simulink subsystem "PvtSubSys_VSM_LCKIE"  (R2020b)
settings: Solver=VariableStepAuto  StartTime=0.0  StopTime=10.0  RelTol=1e-3
values from neighbouring files (symbols this model uses):
  P_VSM_LCKIE_ClassInput = 0.0    [LCKIE.sldd]
  P_VSM_LCKIE_Laneoffset : value not decoded    [LCKIE.sldd]
  P_VSM_LCKIE_Laneoffset_BP : value not decoded    [LCKIE.sldd]
  P_VSM_LCKIE_LatC_DisOffofLanWidth : value not decoded    [LCKIE.sldd]
  P_VSM_LCKIE_LatC_DisOffofSpd : value not decoded    [LCKIE.sldd]
  P_VSM_LCKIE_LatC_DisSW = 0.0    [LCKIE.sldd]
  P_VSM_LCKIE_LatC_LanWidth : value not decoded    [LCKIE.sldd]
  P_VSM_LCKIE_LATC_LimitDis : value not decoded    [LCKIE.sldd]
  P_VSM_LCKIE_LATC_LimitDis_BP : value not decoded    [LCKIE.sldd]
  P_VSM_LCKIE_LatC_LimitDisEgoToObjSelt = 1.5    [LCKIE.sldd]
  P_VSM_LCKIE_LatC_LimitEgoToOppLane = 0.3    [LCKIE.sldd]
  P_VSM_LCKIE_LatC_maxLimitDisREToLane = 2.5    [LCKIE.sldd]
  P_VSM_LCKIE_LatC_minLimitDisREToLane = 1.2    [LCKIE.sldd]
  P_VSM_LCKIE_LatC_MoveEnableDis = 0.0    [LCKIE.sldd]
  P_VSM_LCKIE_LatC_RESafDis = 0.8    [LCKIE.sldd]
  P_VSM_LCKIE_LatC_SafeDisofLanWidth : value not decoded    [LCKIE.sldd]
  P_VSM_LCKIE_LatC_Spd : value not decoded    [LCKIE.sldd]
  P_VSM_LCKIE_LongC_d1 : value not decoded    [LCKIE.sldd]
  P_VSM_LCKIE_LongC_d2 : value not decoded    [LCKIE.sldd]
  P_VSM_LCKIE_LongC_DetaSpd : value not decoded    [LCKIE.sldd]
  P_VSM_LCKIE_LongC_DirecChangeDis = 20.0    [LCKIE.sldd]
  P_VSM_LCKIE_LongC_FleetOff = 80.0    [LCKIE.sldd]
  P_VSM_LCKIE_LongC_maxDis = 80.0    [LCKIE.sldd]
  P_VSM_LCKIE_LongC_minDis = 50.0    [LCKIE.sldd]
  P_VSM_LCKIE_LongC_ShutDownLongDis = -25.0    [LCKIE.sldd]
  P_VSM_LCKIE_LongC_ShutDownTTC = -4.0    [LCKIE.sldd]
  P_VSM_LCKIE_LongC_Spd : value not decoded    [LCKIE.sldd]
  P_VSM_LCKIE_LongC_toff = 10.0    [LCKIE.sldd]
  P_VSM_LCKIE_OFC_ActDis = 10.0    [LCKIE.sldd]
  P_VSM_LCKIE_OFC_DownDis = 10.0    [LCKIE.sldd]
  P_VSM_LCKIE_OFC_DownTTC = 5.0    [LCKIE.sldd]
  P_VSM_LCKIE_OFC_SafDis = 10.0    [LCKIE.sldd]
  P_VSM_LCKIE_OFC_Toff = 3.0    [LCKIE.sldd]
  P_VSM_LCKIE_ORC_LatDis = 1.8    [LCKIE.sldd]
  P_VSM_LCKIE_ORC_LimitDis1 = -30.0    [LCKIE.sldd]
  P_VSM_LCKIE_ORC_LimitDis2 = -10.0    [LCKIE.sldd]
  P_VSM_LCKIE_ORC_LimitTTC = 10.0    [LCKIE.sldd]
  P_VSM_LCKIE_ORC_LowSpd = -5.0    [LCKIE.sldd]
  P_VSM_LCKIE_POC_Delaytime : value not decoded    [LCKIE.sldd]
  P_VSM_LCKIE_POC_detaSpd : value not decoded    [LCKIE.sldd]
  P_VSM_LCKIE_POC_LimitDis = -15.0    [LCKIE.sldd]
  P_VSM_LCKIE_POC_LimitTTC = 2.0    [LCKIE.sldd]
  P_VSM_LCKIE_State_CurveMax = 0.005    [LCKIE.sldd]
  P_VSM_LCKIE_State_CurveMin = 0.0055555555555555558    [LCKIE.sldd]
  P_VSM_LCKIE_State_detaspd = 1.39    [LCKIE.sldd]
  P_VSM_LCKIE_State_detaspd_enable = 1.0    [LCKIE.sldd]
  P_VSM_LCKIE_State_DriverInputTrqValue_enable = 1.0    [LCKIE.sldd]
  P_VSM_LCKIE_State_ELKObjClc = 1.0    [LCKIE.sldd]
  P_VSM_LCKIE_State_HWASts_disable = 1.0    [LCKIE.sldd]
  P_VSM_LCKIE_State_IEObjClc = 1.0    [LCKIE.sldd]
  P_VSM_LCKIE_State_IFVReady = 1.0    [LCKIE.sldd]
  P_VSM_LCKIE_State_lamb_enable = 1.0    [LCKIE.sldd]
  P_VSM_LCKIE_State_Lanecurve_enable = 1.0    [LCKIE.sldd]
  P_VSM_LCKIE_State_LaneWidth_enable = 1.0    [LCKIE.sldd]
  P_VSM_LCKIE_State_Off2on = 3.0    [LCKIE.sldd]
  P_VSM_LCKIE_State_OppObjClc = 1.0    [LCKIE.sldd]
  P_VSM_LCKIE_STATE_ORCObjenable = 0.0    [LCKIE.sldd]
  P_VSM_LCKIE_State_Vehspeed_enable = 1.0    [LCKIE.sldd]
  P_VSM_LCKIE_State_wiper_enable = 1.0    [LCKIE.sldd]
  P_VSM_LCKIE_tcycle = 0.02    [LCKIE.sldd]
undefined symbols (not defined in the file or in its folder): P_Global_Vehicle_Length_m, P_Global_VehicleWidthMin_m, P_VSM_LSMC_SampleTime, STATE
libraries: simulink x62
(part 4 of 5)

== system PvtSubSys_VSM_LCKIE/LCKIE/Subsystem1/LCKIE_SignalProcess1/IE_POC/Subsystem ==
  Input : Inport
  Add : Sum  Inputs=++++++
  Gain : Gain  Gain=1/6
  Unit Delay{,2,4..6} (5 alike) : UnitDelay  SampleTime=-1  HasFrameUpgradeWarning=on
  Out1 : Outport
  wires:
  Input/1 -> Unit Delay6/1, Unit Delay5/1, Unit Delay/1, Unit Delay4/1, Unit Delay2/1, Add/1
  Add/1 -> Gain/1
  Unit Delay4/1 -> Add/3
  Unit Delay/1 -> Add/4
  Gain/1 -> Out1/1
  Unit Delay6/1 -> Add/6
  Unit Delay2/1 -> Add/2
  Unit Delay5/1 -> Add/5

== matlab function PvtSubSys_VSM_LCKIE/LCKIE/LCKIE_StateMachine/Subsystem1/MATLAB Function ==
  data: DisLimmit input single; Dis output single; slope input single; DisK1 input single
function Dis = fcn(DisLimmit,slope,DisK1)
Dis = DisK1;
if DisLimmit >=0
    if (DisK1 - slope <= DisLimmit )&& (DisLimmit <= DisK1 + slope)
        Dis = DisLimmit;
    elseif DisK1 > DisLimmit - slope
        Dis = Dis - slope;
    elseif DisK1 < DisLimmit - slope
        Dis = Dis + slope;
    end
else
    if (DisK1 - slope <= DisLimmit )&& (DisLimmit <= DisK1 + slope)
        Dis = DisLimmit;        
    elseif DisK1 > DisLimmit + slope
        Dis = Dis - slope;
    elseif DisK1 < DisLimmit + slope
        Dis = Dis + slope;
    end
end

== matlab function PvtSubSys_VSM_LCKIE/LCKIE/Subsystem1/IEStateClc/MATLAB Function1 ==
  data: HWASts input uint8; LCKSts input; LaneChange input boolean; Flg output uint8; reflgK1 input uint8; reflg output uint8
function [Flg,reflg]  = fcn(HWASts,LCKSts,LaneChange,reflgK1)
Flg = uint8(0);
reflg = uint8(0);

if LCKSts == 3   
    Flg = uint8(1);
    if (HWASts == 5 ||HWASts == 6)
        Flg = uint8(0);
        if LaneChange == 1
            Flg = uint8(1);
            reflg = uint8(1);
        end
        if reflgK1 == 1
            Flg = uint8(1);
            reflg = uint8(1);
        end
    end
end

== matlab function PvtSubSys_VSM_LCKIE/LCKIE/Subsystem1/LCKIE_SignalProcess1/IE_LATC/MATLAB Function1 ==
  data: Direct input uint8; latflg input uint8; latmov input single; movdis output single; detaDis output; Dis2Obj input single; ORCID input uint8; SelctID input uint8; ORCReady input uint8; ORCReadyK1 input; IEAct input; limitDis input single; flgK1 input uint8; flg output uint8
function [movdis,detaDis,flg] = fcn(Direct,latflg,latmov,Dis2Obj,ORCID,SelctID,ORCReady,ORCReadyK1,IEAct,limitDis,flgK1)

detaDis = single(0);
movdis = latmov;
flg = uint8(0);
if IEAct==1
    flg = flgK1;
    if ORCReady==0 && (ORCReadyK1==1 ||flgK1==1)
        flg = uint8(1);
    end
    if ORCReady==1 && ORCReadyK1==0 
        flg = uint8(0);
    end
end

if flg==1
    t_s = round((Dis2Obj(ORCID)+Dis2Obj(SelctID))*5)/10;
    if latflg == 1
        if abs(t_s)<latmov
            if Direct==1 && t_s<0
                movdis = latmov +t_s;
            elseif Direct==1 && t_s >0
                movdis = latmov - t_s;
            end
        else
            if Direct==1
                if t_s > 0
                    movdis = latmov;
                else
                    detaDis = abs(t_s + latmov);
                    movdis = limitDis;
                end
            else
                if t_s < 0
                    movdis = latmov;
                else
                    detaDis = abs(t_s - latmov);
                    movdis = limitDis;
                end
            end
        end
    end
end

== matlab function PvtSubSys_VSM_LCKIE/LCKIE/Subsystem1/LCKIE_SignalProcess1/IE_Long/IE_LongClc ==
  data: DirectChange input uint8; LongDis output single; PocFlg output uint8; IEReady output uint8; LongFlg output uint8; CouterOff output uint16; ID output uint8; Counter output uint8; Counter1 output uint16 size=1; Counter2 output uint16 size=1; Counter3 output uint16 size=1; Dx output single; LatFLg input uint8; ObjLatFailFlg input uint8; TTC input single; ObjSelectID input uint8; DetaSpdSelct input single; ObjLongPos input single; ObjID input uint8; POSLaneRObjID input uint8; LongDown input uint8; time_shutdown input single; LongDisClc input single; FleetOff input single; ShutDownTTC input single; ShutDownLongDis input single; minDis input single; maxDis input single; DirecChangeDis input single; t_LongDis input single; t_cycle input single; IEActK1 input boolean; LongFlgK1 input uint8; CouterOffK1 input uint16; IDK1 input uint8; CounterK1 input uint8; Counter1K1 input uint16; Counter2K1 input uint16; Counter3K1 input uint16; DxK1 input single
function [LongDis,PocFlg,IEReady,LongFlg,CouterOff,ID,Counter,Counter1,Counter2,Counter3,Dx] = fcn(DirectChange,LatFLg,ObjLatFailFlg,...
    TTC,ObjSelectID,DetaSpdSelct,ObjLongPos,ObjID,POSLaneRObjID,LongDown,...
    time_shutdown,LongDisClc,FleetOff,ShutDownTTC,ShutDownLongDis,minDis,maxDis,DirecChangeDis,t_LongDis,t_cycle,...
    IEActK1,LongFlgK1,CouterOffK1,IDK1,CounterK1,Counter1K1,Counter2K1,Counter3K1,DxK1)


ID = uint8(0);
ObjRPosLanelong = single(0);
ObjRPosLaneTTC = single(0);
SpdLimit = single(0);
LongFlg = uint8(0);
PocFlg = uint8(0);
IEReady = uint8(0);
Counter = uint8(0);
Counter1 = uint16(0);
Counter2 = uint16(0);
Counter3 = uint16(0);
CouterOff = CouterOffK1;
LongDis = LongDisClc;
Dx = single(0);


if ObjSelectID >0
    Dx = ObjLongPos(ObjSelectID);
    ID = ObjID(ObjSelectID);
end
if ID == IDK1
    SpdLimit = single(-2);
end

if POSLaneRObjID >0
    ObjRPosLanelong =  ObjLongPos(POSLaneRObjID);
    ObjRPosLaneTTC =  TTC(POSLaneRObjID);
end



if IEActK1 < 1
    CouterOff = uint16(0);
    if  LongDis > 0 && ObjSelectID >0
        if LongFlgK1 == 0
            if Dx<= LongDis
                Counter = min(CounterK1+uint8(1),uint8(50));
                if Counter > 10
                    LongFlg = uint8(1);
                end
            end
        else
            if ID == IDK1  %%纵向Flg锁
                LongDis = FleetOff;
                if Dx<= LongDis
                    LongFlg = uint8(1);
                end
            end
        end
    end
else
    if ObjSelectID == 0  %%退出机制
        if IDK1 ~= 0 
            LongFlg = uint8(1);            
            if DxK1 >=20  %%防止目标纵向距离跳变
                CouterOff = uint16(100);
            else
                CouterOff = uint16(time_shutdown /t_cycle);
            end
        else
            PocFlg = uint8(1);
            if POSLaneRObjID > 0  %%常规退出条件
                if ObjRPosLaneTTC < ShutDownTTC && ObjRPosLanelong < ShutDownLongDis
                    LongFlg = uint8(0);
                else
                    LongFlg = uint8(1);
                end
            else
                Counter1 = min((Counter1K1+uint16(1)),uint16(65534));                               
                if Counter1 < CouterOff
                    LongFlg = uint8(1);
                end                
            end
        end
    else
        CouterOff = uint16(time_shutdown /t_cycle);
        d3 = DetaSpdSelct*t_LongDis;
        t_d = min(max(d3,minDis),maxDis);        
        LongDis = t_d;
        if DirectChange ==0
            if Dx<= LongDis  && DetaSpdSelct > SpdLimit
                LongFlg = uint8(1);
            else
                PocFlg = uint8(1); 
                if POSLaneRObjID > 0
                    if ObjRPosLaneTTC < ShutDownTTC && ObjRPosLanelong < ShutDownLongDis
                        LongFlg = uint8(0);
                    else
                        LongFlg = uint8(1);
                    end
                else
                    if IDK1 == 0
                        Counter2 = min(max(Counter1K1,Counter2K1)+uint16(1),uint16(65534));                     
                    else
                        Counter2 = min(Counter2K1+uint16(1),uint16(65534));
                    end
            
                    if Counter2 < CouterOff
                        LongFlg = uint8(1);
                    end                   
                end
            end
        else
            LongDis = LongDis - DirecChangeDis;
            if Dx > LongDis && (TTC(ObjSelectID)>5 || DetaSpdSelct <0)
               PocFlg = uint8(1);
               if POSLaneRObjID > 0
                   if ObjRPosLaneTTC < ShutDownTTC && ObjRPosLanelong < ShutDownLongDis
                       LongFlg = uint8(0);
                   else
                       LongFlg = uint8(1);
                   end
               else
                   if IDK1 == 0
                       Counter3 = min(max(Counter1K1,Counter3K1)+uint16(1),uint16(65534));
                   else
                       Counter3 = min(Counter3K1+uint16(1),uint16(65534));
                   end                 
                   if Counter3 < CouterOff
                       LongFlg = uint8(1);
                   end                  
               end
           else
                LongFlg = uint8(0);
                ID = uint8(254);
           end
        end
    end
end

if LongDown ==1 && PocFlg ==1 
    LongFlg = uint8(0);
end

if IEActK1 == 0
    if LongFlg == 1 && LatFLg == 1
        IEReady = uint8(1);
    end
elseif IEActK1 ==1
    if LongFlg == 1 && ObjLatFailFlg ==0
        IEReady = uint8(1);
    end
end

== matlab function PvtSubSys_VSM_LCKIE/LCKIE/Subsystem1/LCKIE_SignalProcess1/IE_OFC/OFC2 ==
  data: safeDis input single; ActDis input single; Toff input single; T1 input single; Dis1 input single; EgoLong input single; OppLaneFObjID input uint8; DetaSpd input single; TTC input single; ObjLongPos input single; ObjLength input single; ObjSelsctDx output single size=1; OppObjDetaSpd output single size=1; ObjTTC output single; Tset output single; OppObjReady output uint8 size=1; OppObjFail output uint8; OppObjReadyK1 input uint8; OppObjFailK1 input uint8; CounterK1 input uint8; Counter output uint8 size=1; Counter1K1 input uint8; Counter1 output uint8
function [ObjSelsctDx,OppObjDetaSpd,ObjTTC,Tset,OppObjReady,OppObjFail,Counter,Counter1]= fcn(safeDis,ActDis,...
    Toff,T1,Dis1,EgoLong,OppLaneFObjID,DetaSpd,TTC,ObjLongPos,ObjLength,OppObjReadyK1,OppObjFailK1,CounterK1,Counter1K1)



OppObjReady = uint8(0);
ObjSelsctDx = single(0);
Counter = uint8(0);
Counter1 = uint8(0);
OppObjDetaSpd =single(0);
ObjLong = single(0);
ObjTTC=single(0);
Tset = single(0);
OppObjFail = uint8(0);

if OppLaneFObjID > 0
    ObjSelsctDx = single(ObjLongPos(OppLaneFObjID)-single(EgoLong));   
    OppObjDetaSpd = single(DetaSpd(OppLaneFObjID));  
    ObjTTC = TTC(OppLaneFObjID);
    if  ObjLength(OppLaneFObjID) ==0
        ObjLong = single(8);
    else
        ObjLong = max(min(ObjLength(OppLaneFObjID),single(20)),single(8));
    end

end

if OppLaneFObjID == 0 || ObjSelsctDx>=120
    OppObjReady = uint8(1);
else
   if  OppObjDetaSpd <0 && ObjSelsctDx>=8
        OppObjReady = uint8(1);
   else
       t_h = (ObjLong+2*safeDis)/OppObjDetaSpd;
       Tset =  Toff+t_h;
       if ObjTTC >Tset && ObjSelsctDx > ActDis
           OppObjReady = uint8(1);
       end
   end
end

if OppLaneFObjID > 0 && OppObjDetaSpd >0
  if (ObjTTC>0 && ObjTTC <T1)|| ObjSelsctDx < Dis1
      OppObjFail = uint8(1);
  end
end
    
if OppObjReady~= OppObjReadyK1
    Counter = min(CounterK1+uint8(1),uint8(20));
    if Counter < 15
        OppObjReady = OppObjReadyK1;
    end
end

if OppObjFail~= OppObjFailK1
    Counter1 = min(Counter1K1+uint8(1),uint8(20));
    if Counter1 < 15
        OppObjFail= OppObjFailK1;
    end
end

== matlab function PvtSubSys_VSM_LCKIE/LCKIE/Subsystem1/LCKIE_SignalProcess1/IE_ORC/ORC ==
  data: Dis1 input single; Dis2 input single; minTTC input single; LatDis input single; LowSpd input single; ObjSelsctTTC output single; OppLaneRObjID input uint8; ObjSelsctDx output single; OppObjLatDis output; OppObjSpd output single; DetaSpd input single; TTC input single; DisEgo2Obj input single; ObjLongPos input single; OppREARObjReadyK1 input uint8; CouterK1 input uint8; OppREARObjReady output uint8; Couter output uint8
function [ObjSelsctTTC,ObjSelsctDx,OppObjLatDis,OppObjSpd,...
    OppREARObjReady,Couter]= fcn(Dis1,Dis2,minTTC,LatDis,LowSpd,OppLaneRObjID,...
    DetaSpd,TTC,DisEgo2Obj,ObjLongPos,OppREARObjReadyK1,CouterK1)



OppREARObjReady = uint8(0);
ObjSelsctDx = single(0);
OppObjSpd =single(0);
ObjSelsctTTC = single(0);
OppObjLatDis = single(0);
Couter = uint8(0);


if OppLaneRObjID > 0
    ObjSelsctDx = single(ObjLongPos(OppLaneRObjID));   
    OppObjLatDis = abs(single(DisEgo2Obj(OppLaneRObjID)));  
    OppObjSpd = single(DetaSpd(OppLaneRObjID));
    ObjSelsctTTC = single(TTC(OppLaneRObjID));
end
if OppLaneRObjID == 0 
    OppREARObjReady = uint8(1);
else
    if OppObjSpd < 0  && OppObjSpd > LowSpd 
        if ObjSelsctDx < Dis1 && ObjSelsctTTC < minTTC && OppObjLatDis > LatDis
            OppREARObjReady = uint8(1);
        end
    else
        if ObjSelsctDx < Dis2
            OppREARObjReady = uint8(1);
        end
    end
end

if OppREARObjReady ~= OppREARObjReadyK1
    Couter = min(CouterK1 +uint8(1),uint8(15));
    if Couter<10
        OppREARObjReady = OppREARObjReadyK1;
    end
end

== matlab function PvtSubSys_VSM_LCKIE/LCKIE/Subsystem1/LCKIE_SignalProcess1/IE_OS/OS ==
  data: IEACTK1 input boolean; IEState input uint8; ObjNum input uint8; t_Ego2Left input single; t_Ego2Right input single; ObjID input uint8; OppFObjID output uint8; ObjLongPos input single; ObjLatPos input single; ObjWidth input single; ObjFuType input uint8; ObjVx input single; ObjClass input uint8; VheSpd_ms input single; C_valid input boolean; C_A0 input single; C_A1 input single; C_A2 input single; C_A3 input single; L_valid input boolean; L_A0 input single; L_A1 input single; L_A2 input single; L_A3 input single; R_valid input boolean; R_A0 input single; R_A1 input single; R_A2 input single; R_A3 input single; ObjIDSelectK1 input uint8; CouterK1 input uint8; Couter1K1 input uint8; OppRObjID output uint8; POSRObjID output uint8; DisEgo2ObjSelect output single; DisEgoToObj output; DetaSpdSelect output single; DisEgo2OppLane output single; DetaSpd output single; ObjLane output uint8; TTC output single; ObjSelectID output uint8; ObjIDSelect output uint8; Couter output uint8; Couter1 output uint8
function [OppFObjID,OppRObjID,POSRObjID,DisEgo2ObjSelect,DisEgoToObj,DetaSpdSelect,DisEgo2OppLane,DetaSpd,ObjLane,TTC,...
    ObjSelectID,ObjIDSelect,Couter,Couter1] = fcn(IEACTK1,IEState,ObjNum,t_Ego2Left,t_Ego2Right,ObjID,...
    ObjLongPos,ObjLatPos,ObjWidth,ObjFuType,ObjVx,ObjClass,VheSpd_ms,C_valid,C_A0,C_A1,C_A2,C_A3,...
    L_valid,L_A0,L_A1,L_A2,L_A3,R_valid,R_A0,R_A1,R_A2,R_A3,ObjIDSelectK1,CouterK1,Couter1K1)

ObjLane = uint8(zeros(9,1));
DetaSpd = single(zeros(9,1));
TTC = single(255*zeros(9,1));
DisEgoToObj = single(255*zeros(9,1));
OppFObjID = uint8(0);
OppRObjID = uint8(0);
POSRObjID = uint8(0);
DisEgo2ObjSelect = single(0);
DetaSpdSelect =  single(0);
DisEgo2OppLane =  single(0);
ObjSelectID = uint8(0);
ObjIDSelect = uint8(0);
Couter = uint8(0);
Couter1 = uint8(0);

minLFObjDis = single(255);
minRFObjDis = single(255);
minEgoFDis = single(255);
minLFTruckDis = single(255);
minRFTruckDis = single(255);
minLRDis = single(255);
minRRDis = single(255);
minLFObjID = uint8(0);
minRFObjID = uint8(0);
minEgoFID = uint8(0);
minLFTruckID = uint8(0);
minRFTruckID = uint8(0);
minLRID = uint8(0);
minRRID = uint8(0);

for i=1:ObjNum
    %%
    if ObjID(i) == ObjIDSelectK1
        outoff = single(3.5);
        long1 = single(-110);
        long2 = single(130);
        LongSt = single(0);
        DirectSpd = single(-0.65);
    else
        outoff = single(3.3);
        long1 = single(-100);
        long2 = single(120);
        LongSt = single(1);
        DirectSpd = single(-0.25);
    end
    %% 目标属性提取，后方目标针对弯道情况，借用LM相关位置进行分类
    t_x = ObjLongPos(i);
    t_y = ObjLatPos(i);
    t_w = ObjWidth(i)/2;
    if ObjID(i) >0 && t_x >long1 &&  t_x < long2 && ObjFuType(i)~=2
        if t_x >LongSt  %%目标前后位置区分
            ObjLongSts = uint8(1);
        else
            ObjLongSts = uint8(2);
        end
        DetaSpd(i)= -ObjVx(i);
        absObjSpd = single(VheSpd_ms + ObjVx(i)); %%目标运动方向区分
        if absObjSpd > DirectSpd
            ObjMovDir = 1;
        else
            ObjMovDir = 2;
        end
        if abs(ObjVx(i)) > 0.001 %%TTC计算
            TTC(i) = -t_x/ObjVx(i);
        end
        if C_valid >0 && L_valid > 0 && R_valid > 0
            t_Cy = C_A0+C_A1*t_x+C_A2*t_x^2+C_A3*t_x^3;
            if t_y>t_Cy
                t_side = uint8(1); %% Obj in the left of ego vhicle
            else
                t_side = uint8(2);
            end
            if t_side == 1
                t_Ly = L_A0+L_A1*t_x+L_A2*t_x^2+L_A3*t_x^3;
                kL = L_A1+2*L_A2*t_x+3*L_A3*t_x^2;
                t_Lk = sqrt(kL^2+1);
                ObjEdge2Lane = (t_y - t_Ly)/t_Lk - t_w ;
            else
                t_Ry = R_A0+R_A1*t_x+R_A2*t_x^2+R_A3*t_x^3;
                kR = R_A1+2*R_A2*t_x+3*R_A3*t_x^2;
                t_Rk = sqrt(kR^2+1);
                ObjEdge2Lane = (t_Ry - t_y)/t_Rk - t_w ;
            end
            if ObjLongSts == 1
                t_latDis = ObjEdge2Lane + 0.4;
            else
                t_latDis = abs(ObjEdge2Lane);
            end
            if t_latDis <= 0
                ObjLane(i) = uint8(3);
            elseif t_latDis > 0 && t_latDis <= outoff
                if t_side ==1
                    ObjLane(i) = uint8(1);
                    DisEgoToObj(i) = t_Ego2Left + ObjEdge2Lane;
                elseif t_side ==2
                    ObjLane(i) = uint8(2);
                    DisEgoToObj(i) = -(t_Ego2Right + ObjEdge2Lane);
                end
            end
        end      
       
        if ObjLongSts == 1
            if ObjLane(i) == 1
                if minLFObjDis >= t_x
                    minLFObjDis = t_x;
                    minLFObjID = uint8(i);
                end
            elseif ObjLane(i) == 2
                if minRFObjDis >= t_x
                    minRFObjDis = t_x;
                    minRFObjID = uint8(i);
                end
            elseif ObjLane(i) == 3
                if minEgoFDis > t_x
                    minEgoFDis = t_x;
                    minEgoFID = uint8(i);
                end
            end
        end
        
        if ObjClass(i) ==3 && ObjLongSts == 1 && ObjMovDir == 1
            if ObjLane(i) == 1
                if minLFTruckDis >= t_x
                    minLFTruckDis = t_x;
                    minLFTruckID = uint8(i);
                end
            elseif ObjLane(i) == 2
                if minRFTruckDis >= t_x
                    minRFTruckDis = t_x;
                    minRFTruckID = uint8(i);
                end
            end
        end
        
        if ObjLongSts == 2 &&ObjMovDir == 1
            if ObjLane(i) == 1
                if minLRDis > abs(t_x)
                    minLRDis = abs(t_x);
                    minLRID = uint8(i);
                end
            elseif ObjLane(i) == 2
                if minRRDis> abs(t_x)
                    minRRDis = abs(t_x);
                    minRRID = uint8(i);
                end
            end
        end
    end
end
%% 主目标筛选，并针对相对速度进行相应延时选择处理
if minLFTruckID>0 && minRFTruckID >0
    t_h = minLFTruckDis - minRFTruckDis;
    if t_h >0
        t_selectID = minRFTruckID;
    else
        t_selectID = minLFTruckID;
    end
elseif minLFTruckID == 0 && minRFTruckID >0
    t_selectID = minRFTruckID;
elseif minLFTruckID > 0 && minRFTruckID == 0
    t_selectID = minLFTruckID;
else
    t_selectID = uint8(0);
end
if t_selectID >0
    if ObjID(t_selectID) == ObjIDSelectK1
        if DetaSpd(t_selectID) > -1.3
            ObjSelectID = t_selectID;
        else
            Couter = min(CouterK1+uint8(1),uint8(6));
            if Couter <5
                ObjSelectID = t_selectID;
            end
        end
    else
        if  DetaSpd(t_selectID) >0.1
            Couter1 = min(Couter1K1+uint8(1),uint8(16));
            if Couter1 >10
                ObjSelectID = t_selectID;
            end
        end
    end
end
%%
if ObjSelectID >0
    if ObjLane(ObjSelectID) == 1   
        DisEgo2OppLane = t_Ego2Right;
        OppFObjID = minRFObjID;
        OppRObjID = minRRID;
        POSRObjID = minLRID;
    elseif ObjLane(ObjSelectID) == 2
        DisEgo2OppLane = t_Ego2Left;
        OppFObjID = minLFObjID;
        OppRObjID = minLRID;
        POSRObjID = minRRID;
    end
else
    if IEACTK1==1
        if IEState == 5
            DisEgo2OppLane = t_Ego2Left;
            OppFObjID = minLFObjID;
            OppRObjID = minLRID;
            POSRObjID = minRRID;
        elseif IEState == 4
            DisEgo2OppLane = t_Ego2Right;
            OppFObjID = minRFObjID;
            OppRObjID = minRRID;
            POSRObjID = minLRID;
        end
    end
end
if ObjSelectID >0
    DisEgo2ObjSelect = abs(DisEgoToObj(ObjSelectID));
    DetaSpdSelect =  DetaSpd(ObjSelectID);
    ObjIDSelect = ObjID(ObjSelectID);
end

== matlab function PvtSubSys_VSM_LCKIE/LCKIE/Subsystem1/LCKIE_SignalProcess1/IE_LATC/LATC ==
  data: LatWarning output uint8; DirectChange output uint8; ObjLatFailFlg output uint8; MovDirct output uint8; LatFLg output uint8; IEActFlgK1 input boolean; ObjSelIDK1 input uint8; ObjSelID input uint8; ObjSelectID input uint8; DisEgo2ObjSelt input single; Ego2OppLane input single; DirctClc input uint8; MoveDis input single; MovDisK1 input single; DisEgo2oObjOff input single; minDisEgoToObjSelt input single; minEgoToOppLane input single; MoveEnableDis input single; MovDirctK1 input uint8; LatMovDis output single; LatFLgK1 input uint8; LatMovDisK1 input single; CounterK1 input uint8; Counter1K1 input uint8; Counter2K1 input uint8; Counter3K1 input uint8; Counter4K1 input uint8; Couter5K1 input uint8; Counter output uint8; Counter1 output uint8; Counter2 output uint8; Counter3 output uint8; Counter4 output uint8; Counter5 output uint8
function [LatWarning,DirectChange,ObjLatFailFlg,MovDirct,LatFLg,...
    LatMovDis,Counter,Counter1,Counter2,Counter3,Counter4,Counter5] = fcn(IEActFlgK1,ObjSelIDK1,ObjSelID,ObjSelectID,...
    DisEgo2ObjSelt,Ego2OppLane,DirctClc,MoveDis,MovDisK1,DisEgo2oObjOff,minDisEgoToObjSelt,minEgoToOppLane,MoveEnableDis,...
    MovDirctK1,LatFLgK1,LatMovDisK1,CounterK1,Counter1K1,Counter2K1,Counter3K1,Counter4K1,Couter5K1)

Counter = uint8(0);
Counter1 = uint8(0);
Counter2 = uint8(0);
Counter3 = uint8(0);
Counter4 = uint8(0);
Counter5 = uint8(0);
LatFLg = uint8(0);
LatMovDis = single(0);
DirectChange = uint8(0);
LatWarning = uint8(0);
ObjLatFailFlg = uint8(0);
MovDirct = DirctClc; 

%%
if ObjSelectID>0
    if DisEgo2ObjSelt < DisEgo2oObjOff
        if LatFLgK1 == 0
            if IEActFlgK1 ==0
                if MoveDis>MoveEnableDis
                    t_h = abs(MoveDis - MovDisK1);
                    if t_h <= 0.2
                        Counter = min(CounterK1+uint8(1),uint8(21));
                        if Counter > 20
                            LatFLg = uint8(1);
                            LatMovDis = MoveDis;
                        end
                    end
                end
            end
        else
            if IEActFlgK1 ==1
                if  MovDirct == MovDirctK1
                    LatFLg = uint8(1);
                    LatMovDis = LatMovDisK1;
                    t_m = (MoveDis - LatMovDisK1);
                    if (t_m>0.1 && DisEgo2ObjSelt < minDisEgoToObjSelt) || (t_m <-0.1 && Ego2OppLane < minEgoToOppLane) %%两车距离太近和车太靠近车道线时，可以改变躲闪距离
                        Counter1 = min(Counter1K1 + uint8(1),uint8(21));
                        if Counter1 > 20
                            LatMovDis = MoveDis;
                        end
                    end
                else
                    LatFLg = uint8(1);
                    LatMovDis = LatMovDisK1;
                    Counter2 = min(Counter2K1 + uint8(1),uint8(21));
                    if Counter2  > 5 %%判断躲闪方向是否更新
                        DirectChange = uint8(1);
                    end
                end
            else
                if ObjSelID == ObjSelIDK1 && MoveDis >0
                    LatFLg = uint8(1);
                    LatMovDis = MoveDis;
                end
            end
        end
    else
        t_offset = min(single(3.5),(2*LatMovDisK1 + DisEgo2oObjOff+ single(0.5)));
        if IEActFlgK1 ==1
            if  MovDirct == MovDirctK1
                if DisEgo2ObjSelt < t_offset
                    LatFLg = uint8(1);
                    LatMovDis = LatMovDisK1;
                else
                    if ObjSelID == ObjSelIDK1                       
                        LatFLg = uint8(1);
                        LatMovDis = LatMovDisK1;
                        Counter3 = min(Counter3K1 + uint8(1),uint8(50));
                        if Counter3 > 30
                            ObjLatFailFlg = uint8(1);
                        end                    
                    end
                end
            else
                LatFLg = uint8(1);
                LatMovDis = LatMovDisK1;
                Counter4 = min(Counter4K1 + uint8(1),uint8(10));
                if Counter4 > 5
                    DirectChange = uint8(1);
                end
            end
        end
    end
else
    if IEActFlgK1 ==1
        LatFLg = uint8(1);
        LatMovDis = LatMovDisK1;
    end
end
%%
if  MovDirct == MovDirctK1 && IEActFlgK1 ==1
    if Ego2OppLane< 0.2
        LatWarning = uint8(1);
        Couter5 = min(Couter5K1+uint8(1),uint8(150));
        if Couter5 < 100
            LatFLg = uint8(1);
            LatMovDis = LatMovDisK1;
        else
            LatFLg = uint8(1);
            LatMovDis = single(0.2);
        end
    end
end

if IEActFlgK1 ==1
    MovDirct = MovDirctK1;
end

== matlab function PvtSubSys_VSM_LCKIE/LCKIE/Subsystem1/LCKIE_SignalProcess1/IE_LATC/LatParm ==
  data: IEState input uint8; MovDirct output uint8; MoveDis output single; DisEgo2ObjOff output; ObjLane input uint8; ObjSelectID input uint8; DisEgo2ObjSelect input; SafeDisoffset input single; DisEgo2ObjOffset input; LRe_Valid input boolean; LRe_A0 input single; LRe_A1 input single; L_Valid input boolean; L_A0 input single; L_A1 input single; RRe_Valid input boolean; RRe_A0 input single; RRe_A1 input single; R_Valid input boolean; R_A0 input single; R_A1 input single; C_Valid input; C_A0 input; HalfEgoWidth input; minDisREToLane input single; maxDisREToLane input single; RESafDis input; CounterK1 input uint8; reflgK1 input uint8; DisREToLane output single; SafeDis output single; Counter output uint8; reflg output uint8
function [MovDirct,MoveDis,DisEgo2ObjOff,DisREToLane,SafeDis,Counter,reflg] = fcn(IEState,ObjLane,ObjSelectID,DisEgo2ObjSelect,SafeDisoffset,DisEgo2ObjOffset,...
    LRe_Valid,LRe_A0,LRe_A1,L_Valid,L_A0,L_A1,RRe_Valid,RRe_A0,RRe_A1,R_Valid,R_A0,R_A1,...
    C_Valid,C_A0,HalfEgoWidth,minDisREToLane,maxDisREToLane,RESafDis,CounterK1,reflgK1)

MovDirct = uint8(0);
MoveDis = single(0);
DisREToLane = single(10);
Counter = uint8(0);
reflg = uint8(0);
SafeDis = single(0.6);
DisEgo2ObjOff = DisEgo2ObjOffset;
%% 躲闪方向判断，计算躲向侧边界与车道线距离
if L_Valid >0 && R_Valid >0 && C_Valid
    if ObjLane(ObjSelectID) == 2 ||IEState == 5
        MovDirct = uint8(1);
        if LRe_Valid >0
            DisREToLane = single(abs((LRe_A0/sqrt(LRe_A1^2+1))-(L_A0/sqrt(L_A1^2+1))));
        end
    end
    if ObjLane(ObjSelectID) == 1||IEState == 4
        MovDirct = uint8(2);
        if RRe_Valid >0
            DisREToLane = single(abs((RRe_A0/sqrt(RRe_A1^2+1))-(R_A0/sqrt(R_A1^2+1))));
        end
    end
    %% 安全距离设定
    SafeDis = SafeDisoffset;
    if DisREToLane < minDisREToLane
        Counter = min((CounterK1+uint8(1)),uint8(15));
        if Counter >10
            reflg = uint8(1);
            SafeDis = single(RESafDis);
        end
    else
        if  reflgK1 ==1 && DisREToLane < maxDisREToLane && (IEState == 4 ||IEState == 5)
            reflg = uint8(1);
            SafeDis = single(RESafDis);
        end
    end
    %% 躲闪距离计算    
    if  DisEgo2ObjSelect < DisEgo2ObjOffset
        d1 = HalfEgoWidth+SafeDis;
        if MovDirct ==1 && L_A0 >d1
            Tar_A0 = L_A0 - d1;
            if Tar_A0 > C_A0
                MoveDis =  Tar_A0 - C_A0;
            end
        elseif MovDirct ==2 && abs(R_A0) >d1
            Tar_A0 = R_A0 + d1;
            if Tar_A0 <C_A0
                MoveDis = C_A0 - Tar_A0;
            end            
        end
        MoveDis = abs(round(MoveDis*10)/10);
    end
end

== matlab function PvtSubSys_VSM_LCKIE/LCKIE/Subsystem1/LCKIE_SignalProcess1/IE_OS/ParameterClc ==
  data: IEACTK1 input boolean; HalfEgoWidth input single; Ego2LeLane output single; L_valid input boolean; L_A0 input single; R_valid input boolean; R_A0 input single; L_A1 input single; R_A1 input single; RoadWidthK1 input single; RoadWCounterK1 input uint8; Ego2RiLane output single; RoadWidth output single; RoadWCounter output uint8
function [Ego2LeLane,Ego2RiLane,RoadWidth,RoadWCounter] = fcn(IEACTK1,HalfEgoWidth,L_valid,L_A0,R_valid,R_A0,L_A1,R_A1,RoadWidthK1,RoadWCounterK1)

RoadWidth = single(0);
Ego2LeLane= single(0);
Ego2RiLane= single(0);
RoadWCounter= uint8(0);


if L_valid == 1 &&  R_valid == 1   
    KL = sqrt(L_A1^2+1);
    KR = sqrt(R_A1^2+1);
    RoadWidth = single(abs(L_A0-R_A0)/(max(KL,KR)));
    RoadWidth = single(0.1*(RoadWidth-RoadWidthK1)+RoadWidthK1);
    Ego2LeLane= abs(L_A0/KL)-HalfEgoWidth;
    Ego2RiLane= abs(R_A0/KR)-HalfEgoWidth;
end

if IEACTK1==1 && (L_valid == 0|| R_valid == 0) 
    RoadWCounter = min((RoadWCounterK1 + uint8(1)),uint8(15));
    if RoadWCounter < 10
        RoadWidth = RoadWidthK1;
    end
end

== matlab function PvtSubSys_VSM_LCKIE/LCKIE/Subsystem1/LCKIE_SignalProcess1/IE_POC/POC ==
  data: POCObjLong output single; POCObjTTC output single; LongDown output uint8; PosID output uint8; PosObjID output uint8; LongPos input single; ObjID input uint8; t_off input single; limitDis input single; TTClimit input single; tcycle input single; IEactFlg input boolean; PosFlg input uint8; TTC input single; POSLaneRObjID input uint8; PosObjIDK1 input uint8; CouterK1 input uint8; Couter output uint8; Couter1K1 input uint16; Couter2K1 input uint8; Couter1 output uint16; Couter2 output uint8 size=1
function [POCObjLong,POCObjTTC,LongDown,PosID,PosObjID,Couter,Couter1,Couter2] = fcn(LongPos,ObjID,t_off,limitDis,TTClimit,...
    tcycle,IEactFlg,PosFlg,TTC,POSLaneRObjID,PosObjIDK1,CouterK1,Couter1K1,Couter2K1)
PosID = uint8(0);
Couter = uint8(0);
LongDown = uint8(0);
Couter1 = uint16(0);
Couter2 = uint8(0);
Couteroff = round(t_off/tcycle);
POCObjLong = single(0);
POCObjTTC = single(0);
PosObjID = uint8(0);

if POSLaneRObjID >0
    POCObjLong = LongPos(POSLaneRObjID);
    POCObjTTC = TTC(POSLaneRObjID);
end


if IEactFlg >0
    if PosFlg ==1
        Couter1 = min(Couter1K1+uint16(1),uint16(65534));     
        if POSLaneRObjID>0
            if PosObjIDK1 == ObjID(POSLaneRObjID)
                LimtDis = limitDis - single(25);
            else
                 LimtDis = limitDis;
            end
                
            if LongPos(POSLaneRObjID)> LimtDis || (TTC(POSLaneRObjID)<TTClimit && TTC(POSLaneRObjID) >0)
                Couter = min(CouterK1+uint8(1),uint8(15));
                if Couter >10
                    PosID = POSLaneRObjID;
                end
            end
        end        
        PosObjID = ObjID(POSLaneRObjID);
       
        if Couter1 > Couteroff && PosID ==0
            Couter2 = min(Couter2K1+uint8(1),uint8(15));
            if Couter2 >10 
                if POSLaneRObjID>0
                    PosID = POSLaneRObjID;
                elseif POSLaneRObjID==0
                    LongDown = uint8(1);
                end
            end
        end
    end
end



%
%
%
%             if LongPos(minPOSLaneRObjID)< limitDis && CouterK1 ==0
%                 minPosID = uint8(0);
%                 Counter1 = Counter1K1+1;
%                 if Counter1 > t_off
%                     if minPOSLaneRObjID >0
%                         minPosID = minPOSLaneRObjID;
%                     else
%                         LongDown = uint8(1);
%                     end
%                 end
%             else
%                 if LongPos(minPOSLaneRObjID)> limitDis
%                     Couter = CouterK1 +1;
%                     if Couter >10
%                         minPosID = minPOSLaneRObjID;
%                     end
%                 end
%             end
% %             if ObjID(minPOSLaneRObjID) == ObjIDSlecK1
% %                 minPosID = minPOSLaneRObjID;
% %             end
%             if DetaSpd(minPOSLaneRObjID)<-1.5
%                 Couter3 = Couter3K1 +1;
%                 if Couter3 >10
%                     minPosID = minPOSLaneRObjID;
%                 end
%             end
%              ObjIDSlec = ObjID(minPosID);
% %         else
% %             Counter2 = Counter2K1+1;
% %                 if Counter2 > t_off
% %                     LongDown = uint8(1);
% %                 end
%         end
%      end
% end

== matlab function PvtSubSys_VSM_LCKIE/LCKIE/Subsystem1/LCKIE_SignalProcess1/IE_POC/POS ==
  data: ObjID input uint8; OvertakeFlg output uint8; ObjSeIDK1 input uint8; ObjSelectID input uint8; DetaSpd input single; IEactFlg input boolean; OvertakeSpd output single; DetaSpdSelctK1 input single
function [OvertakeFlg,OvertakeSpd]  = fcn(ObjID,ObjSeIDK1,ObjSelectID,DetaSpd,IEactFlg,DetaSpdSelctK1)
OvertakeSpd = DetaSpdSelctK1;
OvertakeFlg = uint8(0);
if IEactFlg >0
    if (ObjSeIDK1 ~=0 && ObjSelectID==0) || (ObjSeIDK1 ~= ObjID(ObjSelectID)&& ObjSeIDK1 ~=0)
       OvertakeSpd = DetaSpd;       
       OvertakeFlg = uint8(1);
    end
end
